simulink model "param_ident_online"  (R2025b)
settings: Solver=VariableStepAuto  StartTime=0.0  StopTime=40  RelTol=1e-3
libraries: simulink x4
settings Model: Creator=finnb  LastModifiedBy=trist

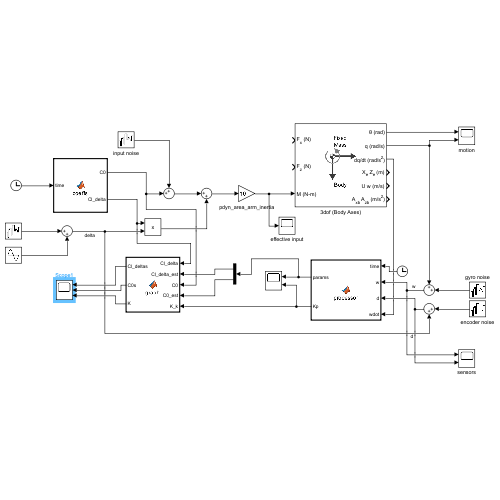
[thumbnail: Simulink's stored preview of the top-level diagram]
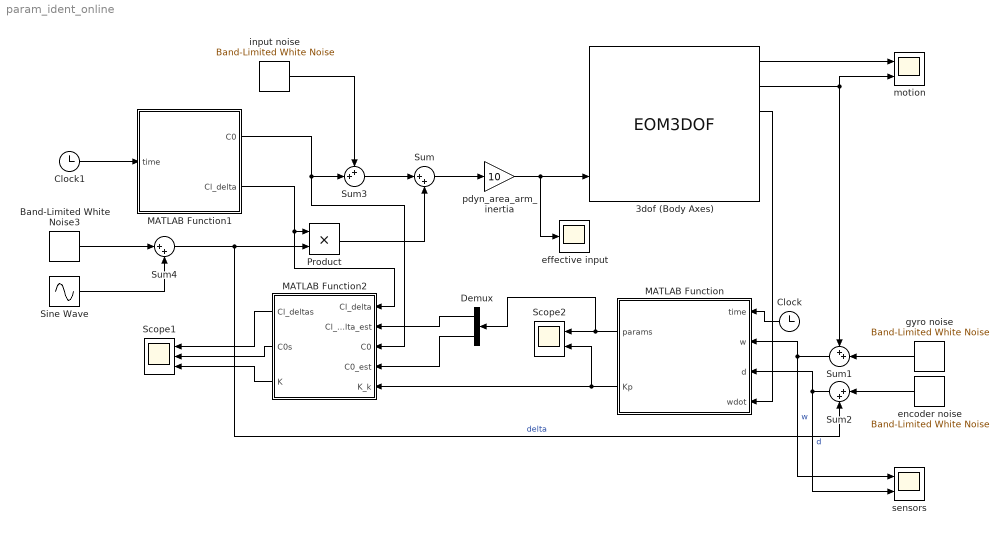
== system param_ident_online ==
  3dof (Body Axes) : EOM3DOF
  Band-Limited White Noise3 : simulink/Sources/Band-Limited White Noise  Cov=[1e-2]  Ts=0.03  seed=[23341]
  Clock : Clock
  Clock1 : Clock
  Demux : Demux  Outputs=2
  MATLAB Function : MATLAB Function  TreatAsAtomicUnit=on
  MATLAB Function1 : MATLAB Function  TreatAsAtomicUnit=on  SystemSampleTime=0.01
  MATLAB Function2 : MATLAB Function  TreatAsAtomicUnit=on  SystemSampleTime=0.01
  Product : Product
  Scope1 : Scope  NumInputPorts=3
      settings: ActiveDisplayYMinimum=0.30388384795953555  ActiveDisplayYMaximum=3.070001445331207  DataLoggingVariableName=ScopeData4
  Scope2 : Scope  NumInputPorts=2
      settings: ActiveDisplayYMinimum=-1  ActiveDisplayYMaximum=1  DataLoggingVariableName=ScopeData2
  Sine Wave : Sin  Frequency=10  Phase=pi/2  SampleTime=0
  Sum : Sum  Inputs=|++
  Sum1 : Sum  Inputs=++|
  Sum2 : Sum  Inputs=|++
  Sum3 : Sum  Inputs=++|
  Sum4 : Sum  Inputs=|++
  effective input : Scope
      settings: ActiveDisplayYMinimum=-1.02773375644536  ActiveDisplayYMaximum=0.770997565307938
  encoder noise : simulink/Sources/Band-Limited White Noise  Cov=[1e-6]  Ts=0.01  seed=[23341]
  gyro noise : simulink/Sources/Band-Limited White Noise  Cov=[1e-7]  Ts=0.01  seed=[23341]
  input noise : simulink/Sources/Band-Limited White Noise  Cov=[1e-6]  Ts=0.2  seed=[23341]
  motion : Scope  NumInputPorts=2
      settings: ActiveDisplayYMinimum=-0.19631545898943475  ActiveDisplayYMaximum=0.622021137740925
  pdyn_area_arm_inertia : Gain  Gain=10
  sensors : Scope  NumInputPorts=2
      settings: ActiveDisplayYMinimum=-0.021581740856872682  ActiveDisplayYMaximum=0.046913425503183052  DataLoggingVariableName=ScopeData3
  wires:
  Sum4/1 -> Product/2, Sum2/2  "delta"
  3dof (Body Axes)/2 -> Sum1/1, motion/2
  Clock/1 -> MATLAB Function/1(time)
  MATLAB Function/1(params) -> Demux/1, Scope2/1
  Sum1/1 -> sensors/1, MATLAB Function/2(w)  "w"
  gyro noise/1 -> Sum1/2
  Sum2/1 -> sensors/2, MATLAB Function/3(d)  "d"
  encoder noise/1 -> Sum2/1
  input noise/1 -> Sum3/1
  pdyn_area_arm_inertia/1 -> effective input/1, 3dof (Body Axes)/3
  Band-Limited White Noise3/1 -> Sum4/1
  Sine Wave/1 -> Sum4/2
  3dof (Body Axes)/1 -> motion/1
  MATLAB Function/2(Kp) -> MATLAB Function2/5(K_k), Scope2/2
  3dof (Body Axes)/3 -> MATLAB Function/4(wdot)
  Sum/1 -> pdyn_area_arm_inertia/1
  Sum3/1 -> Sum/1
  Product/1 -> Sum/2
  MATLAB Function1/2(Cl_delta) -> MATLAB Function2/1(Cl_delta), Product/1
  MATLAB Function1/1(C0) -> MATLAB Function2/3(C0), Sum3/2
  Clock1/1 -> MATLAB Function1/1(time)
  Demux/1 -> MATLAB Function2/2(Cl_delta_est)
  Demux/2 -> MATLAB Function2/4(C0_est)
  MATLAB Function2/1(Cl_deltas) -> Scope1/1
  MATLAB Function2/2(C0s) -> Scope1/2
  MATLAB Function2/3(K) -> Scope1/3

== matlab function param_ident_online/MATLAB Function1 ==
  data: C0 output; time input; Cl_delta output
function [C0, Cl_delta] = coeffs(time)

    persistent Cl_delta_low Cl_delta_high C0_low C0_high Cl_delta_delay C0_delay;
    if isempty(Cl_delta_low)
        Cl_delta_low = 2 * rand - 1; % [-1, 1)
    end
    if isempty(Cl_delta_high)
        Cl_delta_high = 2 * rand + 1; % [1, 3)
    end
    if isempty(C0_low)
        C0_low = - 1 / 10 * rand; % (-0.1, 0)
    end
    if isempty(C0_high)
        C0_high = 1 / 10 * rand; % [0, 0.1)
    end
    if isempty(Cl_delta_delay)
        Cl_delta_delay = rand; % offset the jump
    end
    if isempty(C0_delay)
        C0_delay = rand; % offset jump
    end

    t = time / 40.0;


    

    Cl_delta = Cl_delta_low + (Cl_delta_high - Cl_delta_low) / (1 + exp(-10 * (t - Cl_delta_delay)));
    C0 = C0_low + (C0_high - C0_low) / (1 + exp(-10 * (t - C0_delay)));
end

== matlab function param_ident_online/MATLAB Function ==
  settings: updateMethod=DISCRETE  sampleTime=0.01
  data: time input; w input; params output; d input; Kp output; wdot input
function [params, Kp] = processor(time, w, d, wdot)
    % p : parameters
    % r : regressors
    % w : angular rate measurement
    % d : canard angle measurement / command

    pdyn_area_arm_inertia = 10; % everything in L except coefficients. match with gain in sim

    [params, Kp] = param_estimator_kf(time, w, d, pdyn_area_arm_inertia, wdot);

end

== matlab function param_ident_online/MATLAB Function2 ==
  data: Cl_deltas output; C0s output; Cl_delta input; Cl_delta_est input; C0 input; C0_est input; K_k input; K output
function [Cl_deltas, C0s, K] = graph(Cl_delta, Cl_delta_est, C0, C0_est, K_k)

    Cl_deltas = [Cl_delta, Cl_delta_est];
    C0s = [C0, C0_est];
    K = K_k;
end
